simulink model "punto_5a"  (R2023a)
settings: Solver=VariableStepAuto  StartTime=0.0  StopTime=10.0  RelTol=1e-3
settings Model: Creator=laura  LastModifiedBy=laura

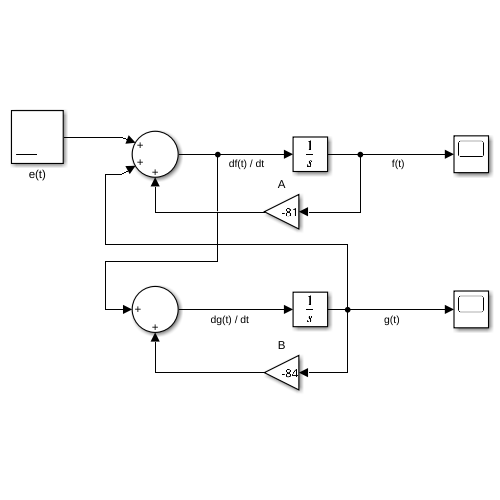
[thumbnail: Simulink's stored preview of the top-level diagram]
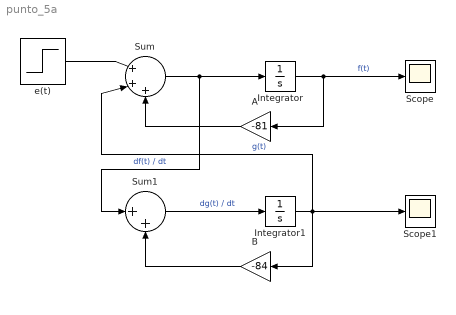
== system punto_5a ==
  A : Gain  Gain=-81
  B : Gain  Gain=-84
  Integrator : Integrator
  Integrator1 : Integrator
  Scope : Scope
  Scope1 : Scope
  Sum : Sum  Inputs=|+++
  Sum1 : Sum  Inputs=|++
  e(t) : Step  SampleTime=0
  wires:
  B/1 -> Sum1/2
  Integrator/1 -> A/1, Scope/1  "f(t)"
  Sum/1 -> Sum1/1, Integrator/1  "df(t) / dt"
  Sum1/1 -> Integrator1/1  "dg(t) / dt"
  e(t)/1 -> Sum/1
  A/1 -> Sum/3
  Integrator1/1 -> B/1, Scope1/1, Sum/2  "g(t)"
